simulink model "DAB"  (R2022a)
settings: Solver=VariableStepAuto  StartTime=0.0  StopTime=10  RelTol=1e-3
libraries: spsMosfetLib x4, spsThyristorLib x4, spsSeriesRLCBranchLib x3, spsVoltageMeasurementLib x2, spsLinearTransformerLib x1, spsDCVoltageSourceLib x1, spspowerguiLib x1
settings Model: Creator=DELL  LastModifiedBy=Asus

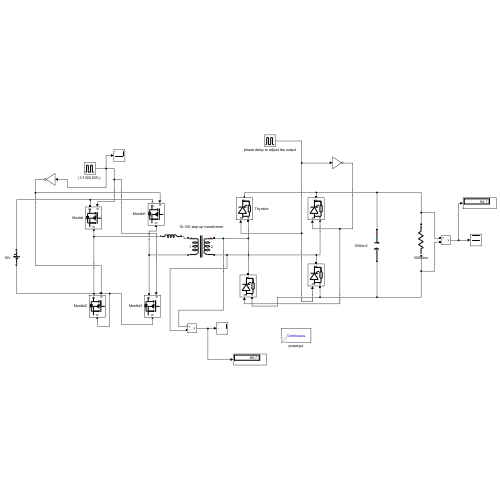
[thumbnail: Simulink's stored preview of the top-level diagram]
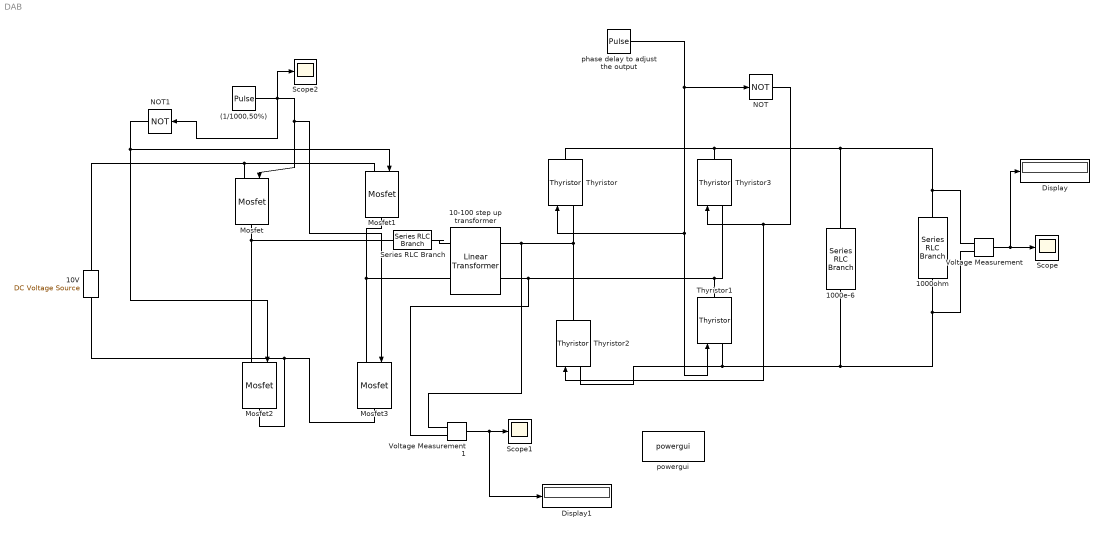
== system DAB ==
  "(1/1000,50%) " : DiscretePulseGenerator  PulseType=Time based  Period=1/1000  PulseWidth=50
  10-100 step up transformer : spsLinearTransformerLib/Linear Transformer  UNITS=pu  NominalPower=[ 1000 1000 ]  winding1="[ 10  0  0 ]"  winding2="[ 100  0  0 ]"  ThreeWindings=off  winding3=[ 315e3 0.002 0.08 ]  RmLm=[ 500 500 ]  Measurements=None  DataType=off
  1000e-6 : spsSeriesRLCBranchLib/Series RLC Branch  LConnTagsString=__new0  RConnTagsString=__new0  BranchType=C  Resistance=1000  Inductance=1e-3  SetiL0=off  InitialCurrent=0  Capacitance=1000e-6  Setx0=off  InitialVoltage=0  Measurements=None
  1000ohm : spsSeriesRLCBranchLib/Series RLC Branch  LConnTagsString=__new0  RConnTagsString=__new0  BranchType=R  Resistance=1000  Inductance=1e-3  SetiL0=off  InitialCurrent=0  Capacitance=1e-6  Setx0=off  InitialVoltage=0  Measurements=None
  10V : spsDCVoltageSourceLib/DC Voltage Source  Amplitude=10  Measurements=None
  Display : Display
  Display1 : Display
  Mosfet{,1..3} (4 alike) : spsMosfetLib/Mosfet  Ron=0.1  Lon=0  Rd=0.01  Vfd=0  IC=0  Rs=1e5  Cs=inf  Measurements=off
  NOT : Logic  Operator=NOT  IconShape=distinctive  AllPortsSameDT=off  OutDataTypeStr=boolean
  NOT1 : Logic  Operator=NOT  IconShape=distinctive  AllPortsSameDT=off  OutDataTypeStr=boolean
  Scope : Scope
  Scope1 : Scope
  Scope2 : Scope
  Series RLC Branch : spsSeriesRLCBranchLib/Series RLC Branch  LConnTagsString=__new0  RConnTagsString=__new0  BranchType=L  Resistance=1  Inductance=30e-6  SetiL0=off  InitialCurrent=0  Capacitance=1e-6  Setx0=off  InitialVoltage=0  Measurements=None
  Thyristor{,1..3} (4 alike) : spsThyristorLib/Thyristor  Ron=0.001  Lon=0  Vf=0.8  IC=0  Rs=500  Cs=250e-9  Measurements=off
  Voltage Measurement : spsVoltageMeasurementLib/Voltage Measurement  PhasorSimulation=off  OutputType=Complex  PSBequivalent=0
  Voltage Measurement1 : spsVoltageMeasurementLib/Voltage Measurement  PhasorSimulation=off  OutputType=Complex  PSBequivalent=0
  phase delay to adjust the output : DiscretePulseGenerator  PulseType=Time based  Period=1/1000  PulseWidth=50  PhaseDelay=0.0834*(1/1000)
  powergui : spspowerguiLib/powergui  Priority=1  SimulationMode=Continuous  SampleTime=50e-6  frequency=60  Iterations=50  frequencyindice=0  Pbase=100e6  ErrMax=1e-4  UnitsV=kV  UnitsW=MW  buscounter=0  FunctionMessages=off  echomessages=off  EnableUseOfTLC=off  CurrentSourceSwitches=off  DisableSnubberDevices=off  DisableRonSwitches=off  DisableVfSwitches=off  DisplayEquations=off  AutomaticDiscreteSolvers=off  SolverType=Tustin/Backward Euler (TBE)  Interpol=off  ExternalGateDelay=off  methode=off  Ts=100  x0status=zero  SPID=on  SwTol=0  HookPort=off  NonlinearTolerance=1e-4  nMaxIteration=100  ContinueOnMaxIteration=off  RestoreLinks=warning  ResistiveCurrentMeasurement=off  Frange=[0:2:500]  Ylog=off  Xlog=on  ShowGrid=off  save=off  variable=ZData  structure=0  ZoomFFT=off  StartTime=0.0  cycles=1  DisplayStyle=1  fundamental=60  FreqAxis=off  MaxFrequency=1000  frequencyindicesteady=1  RmsSteady=1  display=off
  wires:
  Voltage Measurement/1 -> Display/1, Scope/1
  Voltage Measurement1/1 -> Display1/1, Scope1/1
  "(1/1000,50%) "/1 -> NOT1/1, Scope2/1, Mosfet3/1, Mosfet/1
  phase delay to adjust the output/1 -> Thyristor1/1, Thyristor/1, NOT/1
  NOT/1 -> Thyristor2/1, Thyristor3/1
  NOT1/1 -> Mosfet1/1, Mosfet2/1
  connections:
  Mosfet2/LConn1 -- Series RLC Branch/LConn1 -- Mosfet/RConn1
  Mosfet/LConn1 -- 10V/RConn1 -- Mosfet1/LConn1
  Mosfet2/RConn1 -- 10V/LConn1 -- Mosfet3/RConn1
  Mosfet3/LConn1 -- 10-100 step up transformer/LConn2 -- Mosfet1/RConn1
  Thyristor2/RConn1 -- Voltage Measurement1/LConn1 -- 10-100 step up transformer/RConn1 -- Thyristor/LConn1
  Thyristor1/RConn1 -- Thyristor3/LConn1 -- Voltage Measurement1/LConn2 -- 10-100 step up transformer/RConn2
  Thyristor3/RConn1 -- Thyristor/RConn1 -- Voltage Measurement/LConn1 -- 1000ohm/LConn1 -- 1000e-6/LConn1
  Thyristor2/LConn1 -- Voltage Measurement/LConn2 -- 1000ohm/RConn1 -- 1000e-6/RConn1 -- Thyristor1/LConn1
  Series RLC Branch/RConn1 -- 10-100 step up transformer/LConn1
